simulink model "Concatenate2"  (R2017b)
settings: Solver=FixedStepDiscrete  StartTime=0.0  StopTime=10.0  FixedStep=0.200000  RelTol=1e-3  EnableMultiTasking=on
model workspace (MAT data in the model file):
  already_pp = 0
  input_struct.time = [0; 0.2; 0.4; 0.6; 0.8; 1; 1.2; 1.4; 1.6; 1.8; 2; 2.2; 2.4; 2.6; 2.8; 3; 3.2; 3.4; 3.6; 3.8; 4; 4.2; 4.4; 4.6; 4.8; 5; 5.2; 5.4; 5.6; 5.8; 6; 6.2; 6.4; 6.6; 6.8; 7; 7.2; 7.4; 7.6; 7.8; 8; 8.2; 8.4; 8.6; 8.8; 9; 9.2; 9.4; 9.6; 9.8; 10; 10.2; 10.4; 10.6; 10.8; 11; 11.2; 11.4; 11.6; 11.8; 12; 12.2; 12.4; 12.6; 12.8; 13; 13.2; 13.4; 13.6; 13.8; 14; 14.2; 14.4; 14.6; 14.8; 15; 15.2; 15.4; 15.6; 15.8; 16; 16.2; 16.4; 16.6; 16.8; 17; 17.2; 17.4; 17.6; 17.8; 18; 18.2; 18.4; 18.6; 18.8; 19; 19.2; 19.4; 19.6; 19.8]
  input_struct.signals(1).name = 'In1'
  input_struct.signals(1).values = [26.9134575895; 60.523371221; 12.8343482211; 80.7796960178; 86.3114821523; 9.44270570744; 17.8692563362; 36.4950121115; 54.4509179181; 21.9987216848; 23.2196872353; 77.2337138736; 89.7168504921; 2.89571453213; 82.5426562333; 59.3595147348; 98.3045904822; 6.26291447929; 38.7341844794; 20.5245779303; 61.0076411029; 11.8990624587; 81.4867466367; 3.42474960996; 73.9877839811; 7.21150850204; 87.1838635536; 33.6296168259; 28.8927660493; 5.39065335137; 41.1588317805; 36.7410670648; 76.6903077568; 20.1267062487; 71.4315045126; 74.8637819885; 98.7361864603; 70.6608560235; 21.1979727413; 7.41615825596; 53.1648325123; 69.7631834657; 59.1635293614; 58.5009575936; 8.07331814975; 94.8776260547; 85.8301353403; 83.3133456206; 35.5375249455; 97.1712910487; 20.4688027955; 24.9713638681; 32.8189108877; 11.0062423023; 72.767046972; 99.5106192959; 14.2222612344; 20.8624246627; 44.5560862934; 67.8418830317; 26.7620749886; 17.3107842614; 97.7644812595; 45.2382371159; 29.3852441039; 43.7947807121; 28.2118313853; 18.9544959951; 78.9959869246; 83.9558476458; 83.4724218138; 32.3990651852; 57.0025413337; 27.6570908455; 96.5324158361; 61.5832884077; 5.07540964328; 25.4613157766; 60.0300092661; 49.4058730408; 51.9390537179; 74.8128018106; 91.5583320431; 13.4231552552; 53.4769434037; 86.1867232211; 84.5379398429; 71.1024117007; 80.9229499585; 27.6475207319; 26.4303922816; 32.2896700079; 46.2685132092; 32.7975005799; 39.00708295; 60.7241005503; 98.8207463925; 6.67092408639; 86.467043773; 38.355972995]
  input_struct.signals(1).dimensions = 1
  input_struct.signals(2).name = 'In2'
  input_struct.signals(2).values = [7; 12; 4; 90; 2; 93; 30; 78; 31; 88; 25; 30; 24; 45; 22; 47; 53; 12; 20; 15; 79; 83; 49; 81; 32; 49; 100; 96; 88; 77; 47; 97; 8; 77; 69; 7; 44; 30; 60; 66; 71; 72; 4; 63; 77; 58; 62; 59; 37; 8; 80; 47; 59; 49; 2; 47; 58; 66; 66; 65; 97; 11; 20; 87; 99; 35; 71; 77; 81; 47; 48; 32; 32; 93; 84; 56; 84; 90; 89; 60; 36; 49; 80; 9; 2; 57; 39; 68; 18; 15; 7; 6; 14; 32; 76; 27; 39; 23; 65; 59]
  input_struct.signals(2).dimensions = 1
settings Model: Creator=ktrinh  LastModifiedBy=hbourbou
settings OptimizationCC: LifeSpan=inf
settings DebuggingCC: AlgebraicLoopMsg=error  ArtificialAlgebraicLoopMsg=error  SFUnexpectedBacktrackingDiag=warning  SFNoUnconditionalDefaultTransitionDiag=warning  SFExecutionAtInitializationDiag=none
settings HardwareCC: ProdBitPerSizeT=32  ProdBitPerPtrDiffT=32  ProdWordSize=32  ProdHWDeviceType=Specified
settings CodeAppCC: StateflowObjectComments=on
settings GRTTargetCC: TargetLangStandard=C89/C90 (ANSI)  GeneratePreprocessorConditionals=Disable all
settings ConfigComp: CovMetricSettings=dw  CovHtmlReporting=on  CovSaveCumulativeToWorkspaceVar=on  CovSaveSingleToWorkspaceVar=on  CovExternalEMLEnable=off

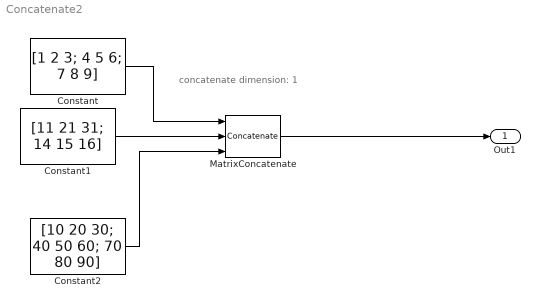
== system Concatenate2 ==
  note: concatenate dimension: 1
  Constant : Constant  Value=[1 2 3; 4 5 6; 7 8 9]
  Constant1 : Constant  Value=[11 21 31; 14 15 16]
  Constant2 : Constant  Value=[10 20 30; 40 50 60; 70 80 90]
  MatrixConcatenate : Concatenate  NumInputs=3  Mode=Multidimensional array
  Out1 : Outport
  wires:
  Constant/1 -> MatrixConcatenate/1
  MatrixConcatenate/1 -> Out1/1
  Constant2/1 -> MatrixConcatenate/3
  Constant1/1 -> MatrixConcatenate/2
